simulink model "adaptiv4"  (Simulink 7.8)
settings: Solver=ode45  StartTime=0.0  StopTime=10.0  RelTol=1e-3
values from neighbouring files (symbols this model uses):
  n_koeff = 32    [adaptiv_4.m]    (also in adaptiv_5.m; adaptiv_6.m)
  ts = (0:length(xs)-1)/250    [adaptiv_4.m]    (also in adaptiv_5.m; adaptiv_6.m)
  Ts = 1/fs    (= 6.25e-05)    [G722_1.m]    (also in adaptiv_2.m = 0.001; adaptiv_3.m = 0.001; adaptiv_4.m = 0.001; adaptiv_5.m = 0.001)
  xs = interp1(0:length(xs)-1, xs, 0:0.25:length(xs)-1,'spline')    [adaptiv_4.m]    (also in adaptiv_5.m; adaptiv_6.m)
libraries: dspadpt3 x1, simulink x1
settings Model: Creator=svenhoffmann  LastModifiedBy=josef  ExtModeAutoUpdateStatusClock=off
settings DataIOCC: SignalLoggingName=sigsOut
settings OptimizationCC: InitFltsAndDblsToZero=on
settings DebuggingCC: SaveWithParameterizedLinksMsg=none  SignalResolutionControl=TryResolveAllWithWarning  SolverPrmCheckMsg=none  MultiTaskDSMMsg=warning  MultiTaskCondExecSysMsg=none  FcnCallInpInsideContextMsg=Use local settings  StrictBusMsg=None
settings HardwareCC: TargetUnknown=on
settings RTWCC: IncludeERTFirstTime=on
settings GRTTargetCC: TargetFcnLib=ansi_tfl_tmw.mat

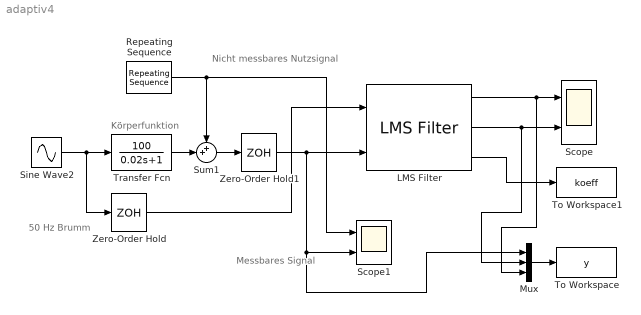
== system adaptiv4 ==
  note: 50 Hz
      | Brumm
  note: Nicht messbares
      | Nutzsignal
  note: Messbares
      | Signal
  note: Körperfunktion
  LMS Filter : dspadpt3/LMS Filter  Algo=Normalized LMS  L=n_koeff  stepflag=Dialog  mu=mu  leakage=1.0  ic=0  Adapt=off  resetflag=None  weights=on  secondCoeffMode=User-defined  secondCoeffWordLength=2  secondCoeffFracLength=15  accum2Mode=User-defined  accum2FracLength=20  prodOutput2Mode=User-defined  prodOutput2FracLength=20  prodOutput3Mode=User-defined  prodOutput3FracLength=20  prodOutput4Mode=User-defined  prodOutput4FracLength=20  quotientMode=User-defined  quotientFracLength=20  roundingMode=Floor  overflowMode=off  addnparflag=off
  Mux : Mux  Inputs=3
  Repeating Sequence : simulink/Sources/Repeating Sequence  rep_seq_t=[ts]  rep_seq_y=[xs]
  Scope : Scope  NumInputPorts=2
      settings: YMin=-7.5~-10  YMax=7.5~10  SaveName=ScopeData2
  Scope1 : Scope  NumInputPorts=2
      settings: YMin=-5~-30  YMax=7.5~30
  Sine Wave2 : Sin  Frequency=2*pi*50  SampleTime=0
  Sum1 : Sum  Inputs=++|  SaturateOnIntegerOverflow=on
  To Workspace : ToWorkspace  VariableName=y  SampleTime=-1  SaveFormat=Array
  To Workspace1 : ToWorkspace  VariableName=koeff  SampleTime=-1  SaveFormat=Array
      settings: MaxDataPoints=1
  Transfer Fcn : TransferFcn  Numerator=[100]  Denominator=[0.02 1]
  Zero-Order Hold : ZeroOrderHold  SampleTime=Ts
  Zero-Order Hold1 : ZeroOrderHold  SampleTime=Ts
  wires:
  Repeating Sequence/1 -> Sum1/1, Scope1/1
  Sine Wave2/1 -> Transfer Fcn/1, Zero-Order Hold/1
  Transfer Fcn/1 -> Sum1/2
  Sum1/1 -> Zero-Order Hold1/1
  LMS Filter/1 -> Scope/1, Mux/3
  LMS Filter/2 -> Scope/2, Mux/2
  LMS Filter/3 -> To Workspace1/1
  Mux/1 -> To Workspace/1
  Zero-Order Hold1/1 -> LMS Filter/2, Scope1/2, Mux/1
  Zero-Order Hold/1 -> LMS Filter/1
